simulink model "mainmodel (2)"  (R2023b)
settings: Solver=FixedStepAuto  StartTime=0.0  StopTime=inf  RelTol=1e-3
libraries: vexarmcortexlib x26, simulink_extras x4, simulink x4, vexcommonlib x3
(part 2 of 2)

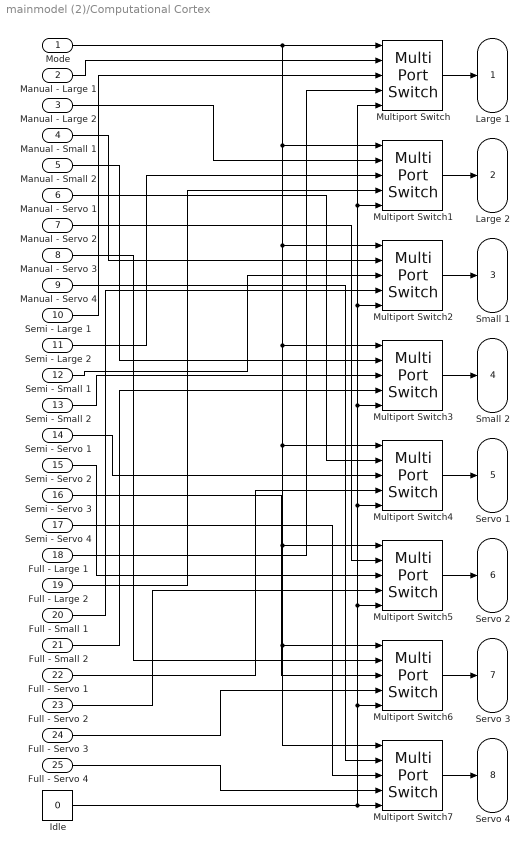
== system mainmodel (2)/Computational Cortex ==
  Mode : Inport
  Manual - Large 1 : Inport  Port=2
  Manual - Large 2 : Inport  Port=3
  Manual - Small 1 : Inport  Port=4
  Manual - Small 2 : Inport  Port=5
  Manual - Servo 1 : Inport  Port=6
  Manual - Servo 2 : Inport  Port=7
  Manual - Servo 3 : Inport  Port=8
  Manual - Servo 4 : Inport  Port=9
  Semi - Large 1 : Inport  Port=10
  Semi - Large 2 : Inport  Port=11
  Semi - Small 1 : Inport  Port=12
  Semi - Small 2 : Inport  Port=13
  Semi - Servo 1 : Inport  Port=14
  Semi - Servo 2 : Inport  Port=15
  Semi - Servo 3 : Inport  Port=16
  Semi - Servo 4 : Inport  Port=17
  Full - Large 1 : Inport  Port=18
  Full - Large 2 : Inport  Port=19
  Full - Small 1 : Inport  Port=20
  Full - Small 2 : Inport  Port=21
  Full - Servo 1 : Inport  Port=22
  Full - Servo 2 : Inport  Port=23
  Full - Servo 3 : Inport  Port=24
  Full - Servo 4 : Inport  Port=25
  Idle : Constant  Value=0
  Multiport Switch{,1..7} (8 alike) : MultiPortSwitch  Inputs=4  SaturateOnIntegerOverflow=off  InputSameDT=off
  Large 1 : Outport
  Large 2 : Outport  Port=2
  Small 1 : Outport  Port=3
  Small 2 : Outport  Port=4
  Servo 1 : Outport  Port=5
  Servo 2 : Outport  Port=6
  Servo 3 : Outport  Port=7
  Servo 4 : Outport  Port=8
  wires:
  Multiport Switch/1 -> Large 1/1
  Multiport Switch1/1 -> Large 2/1
  Multiport Switch3/1 -> Small 2/1
  Multiport Switch2/1 -> Small 1/1
  Multiport Switch5/1 -> Servo 2/1
  Multiport Switch4/1 -> Servo 1/1
  Multiport Switch7/1 -> Servo 4/1
  Multiport Switch6/1 -> Servo 3/1
  Idle/1 -> Multiport Switch/5, Multiport Switch1/5, Multiport Switch2/5, Multiport Switch3/5, Multiport Switch4/5, Multiport Switch5/5, Multiport Switch6/5, Multiport Switch7/5
  Full - Servo 4/1 -> Multiport Switch7/4
  Full - Servo 3/1 -> Multiport Switch6/4
  Full - Servo 2/1 -> Multiport Switch5/4
  Full - Servo 1/1 -> Multiport Switch4/4
  Full - Small 2/1 -> Multiport Switch3/4
  Full - Small 1/1 -> Multiport Switch2/4
  Full - Large 2/1 -> Multiport Switch1/4
  Full - Large 1/1 -> Multiport Switch/4
  Semi - Servo 4/1 -> Multiport Switch7/3
  Semi - Servo 3/1 -> Multiport Switch6/3
  Semi - Servo 2/1 -> Multiport Switch5/3
  Semi - Servo 1/1 -> Multiport Switch4/3
  Semi - Small 2/1 -> Multiport Switch3/3
  Semi - Small 1/1 -> Multiport Switch2/3
  Semi - Large 2/1 -> Multiport Switch1/3
  Semi - Large 1/1 -> Multiport Switch/3
  Manual - Servo 4/1 -> Multiport Switch7/2
  Manual - Servo 3/1 -> Multiport Switch6/2
  Manual - Servo 2/1 -> Multiport Switch5/2
  Manual - Servo 1/1 -> Multiport Switch4/2
  Manual - Small 2/1 -> Multiport Switch3/2
  Manual - Small 1/1 -> Multiport Switch2/2
  Manual - Large 2/1 -> Multiport Switch1/2
  Manual - Large 1/1 -> Multiport Switch/2
  Mode/1 -> Multiport Switch3/1, Multiport Switch4/1, Multiport Switch7/1, Multiport Switch6/1, Multiport Switch5/1, Multiport Switch2/1, Multiport Switch1/1, Multiport Switch/1

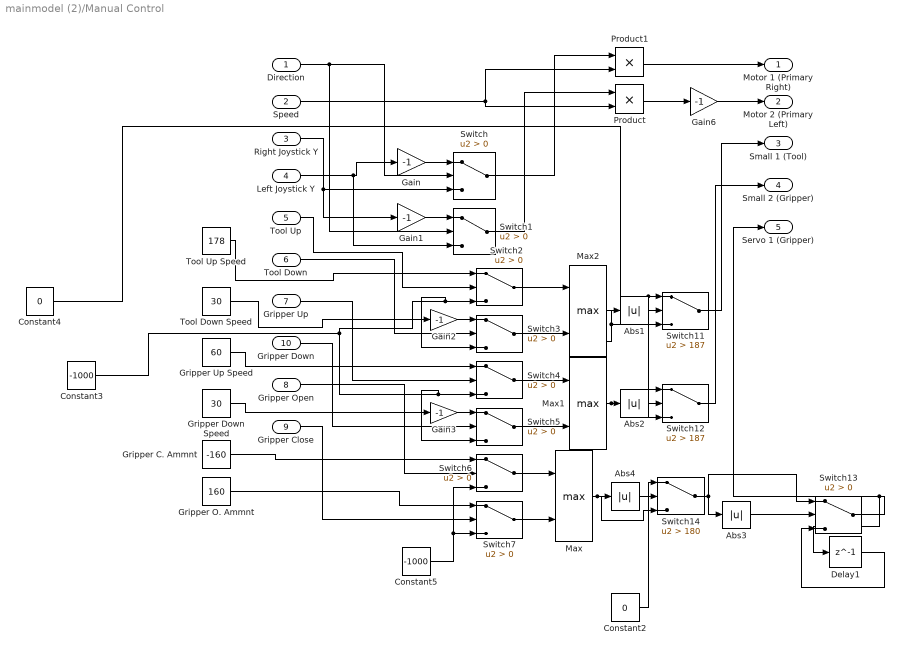
== system mainmodel (2)/Manual Control ==
  Direction : Inport
  Speed : Inport  Port=2
  Right Joystick Y : Inport  Port=3
  Left Joystick Y : Inport  Port=4
  Tool Up : Inport  Port=5
  Tool Down : Inport  Port=6
  Gripper Up : Inport  Port=7
  Gripper Open : Inport  Port=8
  Gripper Close : Inport  Port=9
  Gripper Down : Inport  Port=10
  Abs{1..4} (4 alike) : Abs  SaturateOnIntegerOverflow=off
  Constant2 : Constant  Value=0
  Constant3 : Constant  Value=-1000
  Constant4 : Constant  Value=0
  Constant5 : Constant  Value=-1000
  Delay1 : Delay  DelayLength=1
  Gain{,1..3,6} (5 alike) : Gain  Gain=-1
  Gripper C. Ammnt : Constant  Value=-160
  Gripper Down Speed : Constant  Value=30
  Gripper O. Ammnt : Constant  Value=160
  Gripper Up Speed : Constant  Value=60
  Max : MinMax  Function=max  Inputs=2
  Max1 : MinMax  Function=max  Inputs=2
  Max2 : MinMax  Function=max  Inputs=2
  Product : Product  RndMeth=Zero
  Product1 : Product  RndMeth=Zero
  Switch{,1..7,13} (9 alike) : Switch  Criteria=u2 > Threshold  SaturateOnIntegerOverflow=off  InputSameDT=off
  Switch11 : Switch  Criteria=u2 > Threshold  Threshold=187  SaturateOnIntegerOverflow=off  InputSameDT=off
  Switch12 : Switch  Criteria=u2 > Threshold  Threshold=187  SaturateOnIntegerOverflow=off  InputSameDT=off
  Switch14 : Switch  Criteria=u2 > Threshold  Threshold=180  SaturateOnIntegerOverflow=off  InputSameDT=off
  Tool Down Speed : Constant  Value=30
  Tool Up Speed : Constant  Value=178
  Motor 1 (Primary Right) : Outport
  Motor 2 (Primary Left) : Outport  Port=2
  Small 1 (Tool) : Outport  Port=3
  Small 2 (Gripper) : Outport  Port=4
  Servo 1 (Gripper) : Outport  Port=5
  wires:
  Gripper Close/1 -> Switch7/2
  Gripper Down Speed/1 -> Gain3/1
  Constant4/1 -> Switch12/1, Switch11/1
  Direction/1 -> Switch1/2, Switch/2
  Tool Down/1 -> Switch3/2
  Delay1/1 -> Switch13/3
  Gripper C. Ammnt/1 -> Switch6/1
  Max1/1 -> Switch12/3, Abs2/1
  Abs1/1 -> Switch11/2
  Tool Down Speed/1 -> Gain2/1
  Tool Up/1 -> Switch2/2
  Abs2/1 -> Switch12/2
  Max2/1 -> Abs1/1, Switch11/3
  Gain3/1 -> Switch5/1
  Constant3/1 -> Switch3/3, Switch2/3, Switch5/3, Switch4/3
  Switch6/1 -> Max/1
  Constant2/1 -> Switch14/1
  Switch13/1 -> Servo 1 (Gripper)/1, Delay1/1
  Gain2/1 -> Switch3/1
  Left Joystick Y/1 -> Switch1/3, Gain/1
  Switch/1 -> Product1/1
  Switch11/1 -> Small 1 (Tool)/1
  Gripper Down/1 -> Switch5/2
  Gripper Open/1 -> Switch6/2
  Tool Up Speed/1 -> Switch2/1
  Gripper Up/1 -> Switch4/2
  Switch12/1 -> Small 2 (Gripper)/1
  Switch7/1 -> Max/2
  Speed/1 -> Product/2, Product1/2
  Switch4/1 -> Max1/1
  Switch2/1 -> Max2/1
  Gripper O. Ammnt/1 -> Switch7/1
  Gripper Up Speed/1 -> Switch4/1
  Switch5/1 -> Max1/2
  Gain1/1 -> Switch1/1
  Switch3/1 -> Max2/2
  Right Joystick Y/1 -> Switch/3, Gain1/1
  Switch1/1 -> Product/1
  Gain/1 -> Switch/1
  Abs3/1 -> Switch13/2
  Constant5/1 -> Switch6/3, Switch7/3
  Max/1 -> Switch14/3, Abs4/1
  Abs4/1 -> Switch14/2
  Switch14/1 -> Abs3/1, Switch13/1
  Product/1 -> Gain6/1
  Gain6/1 -> Motor 2 (Primary Left)/1
  Product1/1 -> Motor 1 (Primary Right)/1

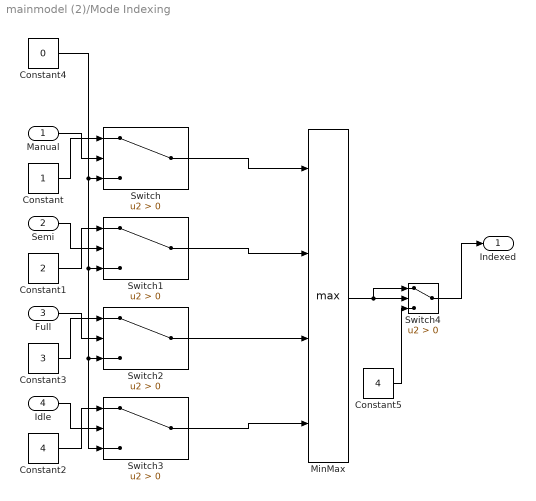
== system mainmodel (2)/Mode Indexing ==
  Manual : Inport
  Semi : Inport  Port=2
  Full : Inport  Port=3
  Idle : Inport  Port=4
  Constant : Constant
  Constant1 : Constant  Value=2
  Constant2 : Constant  Value=4
  Constant3 : Constant  Value=3
  Constant4 : Constant  Value=0
  Constant5 : Constant  Value=4
  MinMax : MinMax  Function=max  Inputs=4
  Switch{,1..4} (5 alike) : Switch  Criteria=u2 > Threshold  SaturateOnIntegerOverflow=off  InputSameDT=off
  Indexed : Outport
  wires:
  Switch/1 -> MinMax/1
  Switch1/1 -> MinMax/2
  Switch2/1 -> MinMax/3
  Switch3/1 -> MinMax/4
  Manual/1 -> Switch/2
  Constant/1 -> Switch/1
  Constant1/1 -> Switch1/1
  Semi/1 -> Switch1/2
  Full/1 -> Switch2/2
  Constant3/1 -> Switch2/1
  Constant2/1 -> Switch3/1
  Idle/1 -> Switch3/2
  Constant4/1 -> Switch3/3, Switch2/3, Switch1/3, Switch/3
  MinMax/1 -> Switch4/1, Switch4/2
  Switch4/1 -> Indexed/1
  Constant5/1 -> Switch4/3

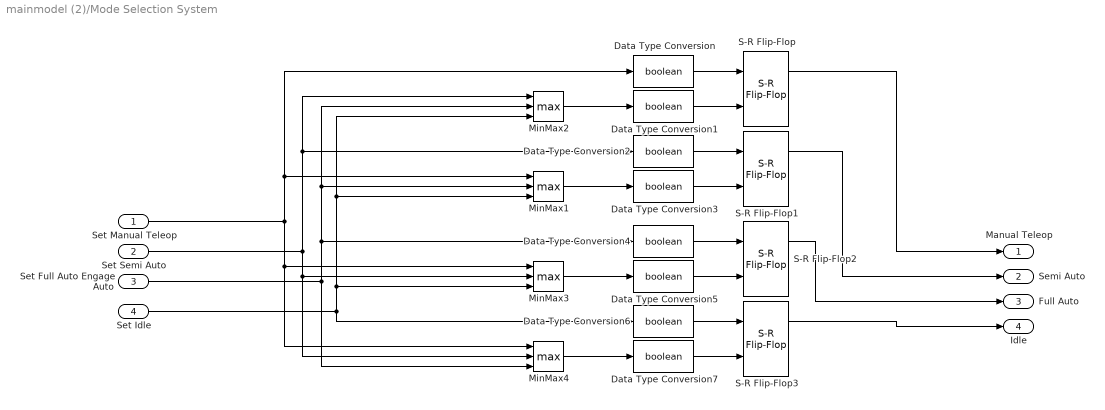
== system mainmodel (2)/Mode Selection System ==
  Set Manual Teleop : Inport
  Set Semi Auto : Inport  Port=2
  Set Full Auto Engage Auto : Inport  Port=3
  Set Idle : Inport  Port=4
  Data Type Conversion{,1..7} (8 alike) : DataTypeConversion  OutDataTypeStr=boolean  ConvertRealWorld=Stored Integer (SI)  SaturateOnIntegerOverflow=off  RndMeth=Floor
  MinMax{1..4} (4 alike) : MinMax  Function=max  Inputs=3
  S-R Flip-Flop{,1..3} (4 alike) : simulink_extras/Flip Flops/S-R Flip-Flop  initial_condition=0
  Manual Teleop : Outport
  Semi Auto : Outport  Port=2
  Full Auto : Outport  Port=3
  Idle : Outport  Port=4
  wires:
  Set Semi Auto/1 -> MinMax3/2, MinMax4/2, MinMax2/1, Data Type Conversion2/1
  Set Full Auto Engage Auto/1 -> MinMax4/3, MinMax1/2, MinMax2/2, Data Type Conversion4/1
  Set Idle/1 -> Data Type Conversion6/1, MinMax3/3, MinMax1/3, MinMax2/3
  S-R Flip-Flop/1 -> Manual Teleop/1
  Data Type Conversion/1 -> S-R Flip-Flop/1
  Data Type Conversion1/1 -> S-R Flip-Flop/2
  MinMax2/1 -> Data Type Conversion1/1
  Set Manual Teleop/1 -> Data Type Conversion/1, MinMax1/1, MinMax3/1, MinMax4/1
  Data Type Conversion2/1 -> S-R Flip-Flop1/1
  MinMax1/1 -> Data Type Conversion3/1
  S-R Flip-Flop1/1 -> Semi Auto/1
  Data Type Conversion3/1 -> S-R Flip-Flop1/2
  Data Type Conversion4/1 -> S-R Flip-Flop2/1
  MinMax3/1 -> Data Type Conversion5/1
  S-R Flip-Flop2/1 -> Full Auto/1
  Data Type Conversion5/1 -> S-R Flip-Flop2/2
  Data Type Conversion6/1 -> S-R Flip-Flop3/1
  MinMax4/1 -> Data Type Conversion7/1
  S-R Flip-Flop3/1 -> Idle/1
  Data Type Conversion7/1 -> S-R Flip-Flop3/2

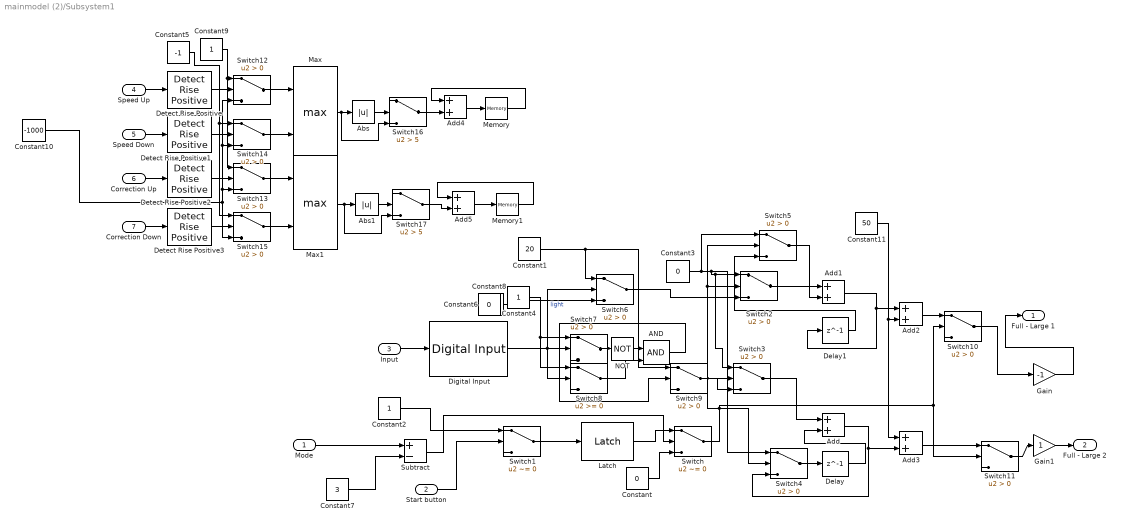
== system mainmodel (2)/Subsystem1 ==
  " Mode" : Inport
  Start button : Inport  Port=2
  Input : Inport  Port=3
  Speed Up : Inport  Port=4
  Speed Down : Inport  Port=5
  Correction Up : Inport  Port=6
  Correction Down : Inport  Port=7
  AND : Logic  IconShape=distinctive  AllPortsSameDT=off  OutDataTypeStr=boolean
  Abs : Abs  SaturateOnIntegerOverflow=off
  Abs1 : Abs  SaturateOnIntegerOverflow=off
  Add{,1..5} (6 alike) : Sum
  Constant{,3,6,8} (4 alike) : Constant  Value=0
  Constant1 : Constant  Value=20
  Constant10 : Constant  Value=-1000
  Constant11 : Constant  Value=50
  Constant2 : Constant
  Constant4 : Constant
  Constant5 : Constant  Value=-1
  Constant7 : Constant  Value=3
  Constant9 : Constant
  Delay : Delay  DelayLength=1
  Delay1 : Delay  DelayLength=1
  Detect Rise Positive{,1..3} (4 alike) : simulink/Logic and Bit Operations/Detect Rise Positive  vinit=0  OutDataTypeStr=boolean
  Digital Input : vexarmcortexlib/Sensors/Digital Input  inChan=1  SimulationIn=on  SampleTime=0.2
  Gain : Gain  Gain=-1
  Gain1 : Gain
  Latch : vexcommonlib/Latch  output0=off  BlockPlatform=vexarmcortex
      settings: LibrarySourceBlock=vexarmcortexlib/Utilities/Latch
  Max : MinMax  Function=max  Inputs=2
  Max1 : MinMax  Function=max  Inputs=2
  Memory : Memory
  Memory1 : Memory
  NOT : Logic  Operator=NOT  IconShape=distinctive  AllPortsSameDT=off  OutDataTypeStr=boolean
  Subtract : Sum  Inputs=+-
  Switch : Switch  Criteria=u2 ~= 0  SaturateOnIntegerOverflow=off  InputSameDT=off
  Switch1 : Switch  Criteria=u2 ~= 0  SaturateOnIntegerOverflow=off  InputSameDT=off
  Switch{2..7,9..15} (13 alike) : Switch  Criteria=u2 > Threshold  SaturateOnIntegerOverflow=off  InputSameDT=off
  Switch16 : Switch  Criteria=u2 > Threshold  Threshold=5  SaturateOnIntegerOverflow=off  InputSameDT=off
  Switch17 : Switch  Criteria=u2 > Threshold  Threshold=5  SaturateOnIntegerOverflow=off  InputSameDT=off
  Switch8 : Switch  SaturateOnIntegerOverflow=off  InputSameDT=off
  Full - Large 1 : Outport
  Full - Large 2 : Outport  Port=2
  wires:
  Memory/1 -> Add4/1
  Digital Input/1 -> Switch8/2, Switch6/2, Switch7/2  "light"
  Delay1/1 -> Switch5/3
  Delay/1 -> Add/2
  Add1/1 -> Add2/1, Delay1/1
  Add/1 -> Switch4/3, Add3/2
  Constant/1 -> Switch/3
  Constant2/1 -> Switch1/1
  Latch/1 -> Switch/1
  Start button/1 -> Switch1/2
  Switch1/1 -> Latch/1
  Switch2/1 -> Add1/1
  Switch9/1 -> Switch3/3
  Switch/1 -> Switch11/2, Switch10/2, Switch5/2, Switch2/2, Switch3/2, Switch4/2
  Constant3/1 -> Switch5/1, Switch4/1, Switch2/1, Switch3/1
  Switch3/1 -> Add/1
  Switch4/1 -> Delay/1
  Switch5/1 -> Add1/2
  Input/1 -> Digital Input/1
  Switch7/1 -> NOT/1
  NOT/1 -> AND/1
  Switch8/1 -> AND/2
  AND/1 -> Switch9/2
  Memory1/1 -> Add5/1
  Switch6/1 -> Switch2/3
  Constant6/1 -> Switch6/3
  Constant4/1 -> Switch8/1, Switch7/1
  Subtract/1 -> Switch/2
  " Mode"/1 -> Subtract/1
  Constant7/1 -> Subtract/2
  Add2/1 -> Switch10/1
  Add3/1 -> Switch11/1
  Switch10/1 -> Gain/1
  Gain/1 -> Full - Large 1/1
  Switch11/1 -> Gain1/1
  Gain1/1 -> Full - Large 2/1
  Speed Up/1 -> Detect Rise Positive/1
  Speed Down/1 -> Detect Rise Positive1/1
  Correction Up/1 -> Detect Rise Positive2/1
  Correction Down/1 -> Detect Rise Positive3/1
  Detect Rise Positive/1 -> Switch12/2
  Detect Rise Positive2/1 -> Switch13/2
  Detect Rise Positive1/1 -> Switch14/2
  Detect Rise Positive3/1 -> Switch15/2
  Constant9/1 -> Switch13/1, Switch12/1
  Constant5/1 -> Switch15/1, Switch14/1
  Switch14/1 -> Max/2
  Switch12/1 -> Max/1
  Constant10/1 -> Switch15/3, Switch13/3, Switch14/3, Switch12/3
  Switch13/1 -> Max1/1
  Switch15/1 -> Max1/2
  Add5/1 -> Memory1/1
  Add4/1 -> Memory/1
  Max/1 -> Switch16/3, Abs/1
  Abs/1 -> Switch16/2
  Max1/1 -> Switch17/3, Abs1/1
  Abs1/1 -> Switch17/2
  Switch16/1 -> Add4/2
  Switch17/1 -> Add5/2
  Constant1/1 -> Switch9/1, Switch6/1
  Constant11/1 -> Add3/1, Add2/2
